simulink model "Question_8_SL"  (R2017a)
settings: Solver=VariableStepAuto  StartTime=0.0  StopTime=7  RelTol=1e-3
settings Model: Creator=berthj01  LastModifiedBy=vonl01

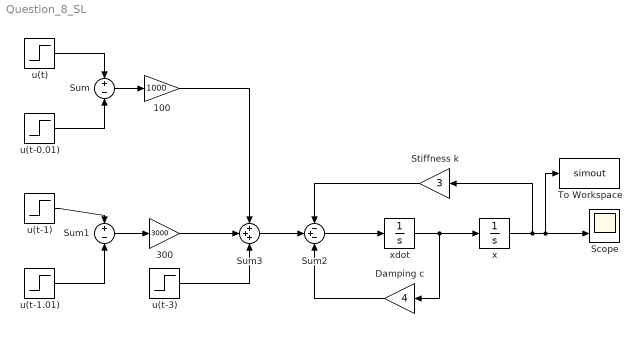
== system Question_8_SL ==
  100 : Gain  Gain=1000
  300 : Gain  Gain=3000
  Damping c : Gain  Gain=4
  Scope : Scope  NumInputPorts=2
  Stiffness k : Gain  Gain=3
  Sum : Sum  Inputs=+-
  Sum1 : Sum  Inputs=+-
  Sum2 : Sum  Inputs=-+-
  Sum3 : Sum  Inputs=+++
  To Workspace : ToWorkspace  VariableName=simout  SampleTime=-1
  u(t) : Step  Time=0  SampleTime=0
  u(t-0.01) : Step  Time=.001  SampleTime=0
  u(t-1) : Step  SampleTime=0
  u(t-1.01) : Step  Time=1.001  SampleTime=0
  u(t-3) : Step  Time=3  SampleTime=0
  x : Integrator
  xdot : Integrator
  wires:
  u(t-0.01)/1 -> Sum/2
  u(t)/1 -> Sum/1
  Sum/1 -> 100/1
  u(t-1)/1 -> Sum1/1
  u(t-1.01)/1 -> Sum1/2
  Sum1/1 -> 300/1
  300/1 -> Sum3/2
  100/1 -> Sum3/1
  u(t-3)/1 -> Sum3/3
  Sum3/1 -> Sum2/2
  Sum2/1 -> xdot/1
  xdot/1 -> Damping c/1, x/1
  x/1 -> To Workspace/1, Scope/2, Stiffness k/1
  Stiffness k/1 -> Sum2/1
  Damping c/1 -> Sum2/3
